simulink model "model"  (R2024a)
settings: Solver=FixedStepAuto  StartTime=0.0  StopTime=100  FixedStep=0.01  RelTol=1e-3
undefined symbols (not defined in the file or in its folder): e0_0, e1_0, e2_0, e3_0, q0, Thrust, vec
libraries: sharedtransform x21, sharedutil x4, aerolibsim3d x2, dspsigops x2, shared6dof x1, sim3dlib x1
(part 1 of 2)
settings Model: Creator=bemran  LastModifiedBy=bemran

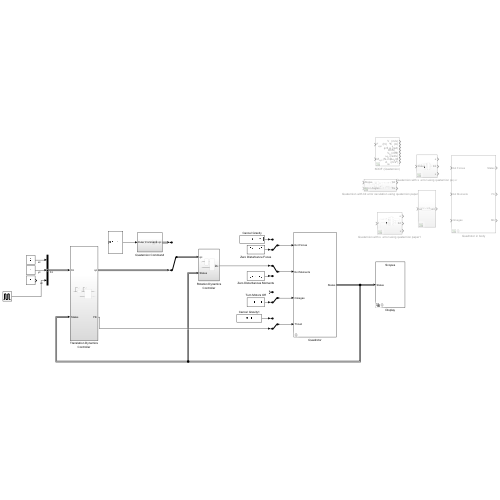
[thumbnail: Simulink's stored preview of the top-level diagram]
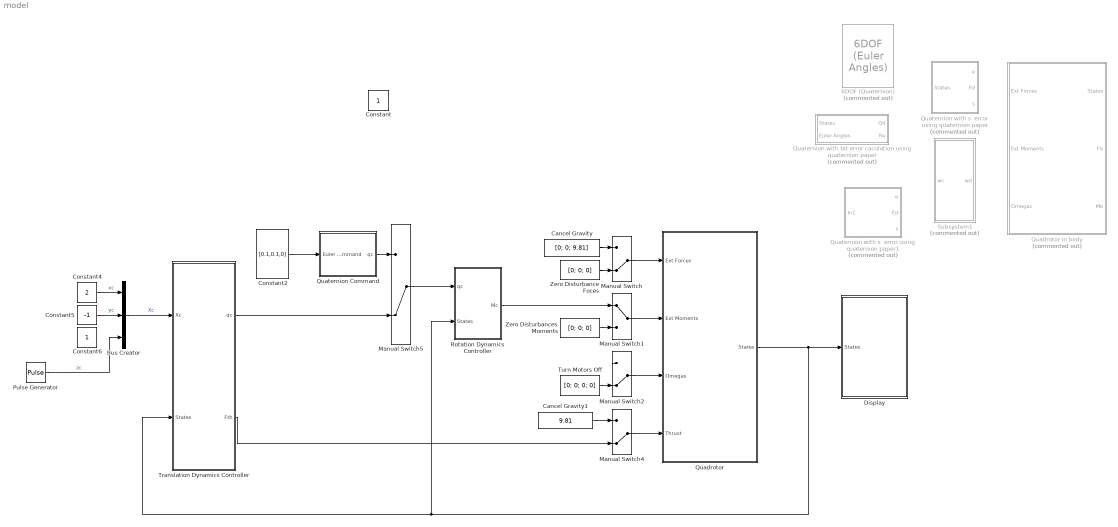
== system model ==
  6DOF (Quaternion) : shared6dof/6DOF (Euler Angles)  Commented=on  units=Metric (MKS)  mtype=Fixed  rep=Quaternion  xme_0=[0 0 0]  Vm_0=[0 0 0]  eul_0=[0 0 0]  pm_0=[0 0 0]  mass_0=1.0  mass_e=0.5  mass_f=2.0  inertia=eye(3)  inertia_e=eye(3)  inertia_f=2*eye(3)  k_quat=1.0  vre_flag=on  abi_flag=off  aMode=0  xme_statename=''  Vm_statename=''  eul_statename=''  quat_statename=''  pm_statename=''  mass_statename=''
      settings: LibrarySourceBlock=aerolib6dof2/6DOF (Quaternion)
  Bus Creator : BusCreator  Inputs=3
  Cancel Gravity : Constant  Value=[0; 0; 9.81]
  Cancel Gravity1 : Constant  Value=9.81
  Constant2 : Constant  Value=[0.1,0.1,0]
  Constant4 : Constant  Value=2
  Constant5 : Constant  Value=-1
  Constant6 : Constant
  Display : Subsystem  Variant=on  VariantControlMode=label  LabelModeActiveChoice=scopes  mask{VChoice=scopes}
      mask prompts: VChoice "Select method of display"
      mask init:
      | vssBlk = gcb;
      | choice = get_param(vssBlk,'VChoice');
      | if strcmp(choice,'animation')
      |     set_param(vssBlk, 'LabelModeActiveChoice', 'animation');
      | else
      |     set_param(vssBlk, 'LabelModeActiveChoice', 'scopes');
      | end
  Manual Switch{,2,4..5} (4 alike) : ManualSwitch  CurrentSetting=0
  Manual Switch1 : ManualSwitch
  Pulse Generator : DiscretePulseGenerator  PulseType=Time based  Amplitude=4  Period=20  PulseWidth=50
  Quadrotor : Subsystem  mask{VChoice=Thrust, mass=1, InertiaMatrix=eye(3)*0.1, thrust_coff=1, drag_coff=0.1, arm_length=0.3, VelocityBodyInitialValues=zeros(3,1), PositionReferenceInitialValues=zeros(3,1), OmegaInitialValues=zeros(3,1), EulerInitialValues=zeros(3,1)}
      mask prompts: VChoice "Select method of applying forces"; InertiaMatrix "Inertia Matrix"; thrust_coff "Thrust Coefficient"; drag_coff "Drag Coefficient"; arm_length "Arm Length"; VelocityBodyInitialValues "Velocity Body Initial Values"; PositionReferenceInitialValues "Position Reference Initial Values"; OmegaInitialValues "Omega Initial Values"; EulerInitialValues "Euler Initial Values"
      mask TypeOptions VChoice: Applied Forces in Body frame/VChoice
      mask TypeOptions mass: 6DOF NED Mixed/mass
      mask TypeOptions InertiaMatrix: 6DOF NED Mixed/InertiaMatrix
      mask TypeOptions thrust_coff: Mixer/thrust_coff
      mask TypeOptions drag_coff: Mixer/drag_coff
      mask TypeOptions arm_length: Mixer/arm_length
      mask TypeOptions VelocityBodyInitialValues: 6DOF NED Mixed/VelocityBodyInitialValues
      mask TypeOptions PositionReferenceInitialValues: 6DOF NED Mixed/PositionReferenceInitialValues
      mask TypeOptions OmegaInitialValues: 6DOF NED Mixed/OmegaInitialValues
      mask TypeOptions EulerInitialValues: 6DOF NED Mixed/EulerInitialValues
  Quadrotor in body : Subsystem  Commented=on  mask{VChoice=Thrust, mass=1, InertiaMatrix=eye(3)*0.1, thrust_coff=1, drag_coff=0.1, arm_length=0.3, VelocityBodyInitialValues=zeros(3,1), PositionReferenceInitialValues=zeros(3,1), OmegaInitialValues=zeros(3,1), EulerInitialValues=zeros(3,1)}
      mask prompts: VChoice "Select method of applying forces"; InertiaMatrix "Inertia Matrix"; thrust_coff "Thrust Coefficient"; drag_coff "Drag Coefficient"; arm_length "Arm Length"; VelocityBodyInitialValues "Velocity Body Initial Values"; PositionReferenceInitialValues "Position Reference Initial Values"; OmegaInitialValues "Omega Initial Values"; EulerInitialValues "Euler Initial Values"
      mask TypeOptions VChoice: Applied Forces in Body frame/VChoice
      mask TypeOptions mass: 6DOF NED Mixed/mass
      mask TypeOptions InertiaMatrix: 6DOF NED Mixed/InertiaMatrix
      mask TypeOptions thrust_coff: Mixer/thrust_coff
      mask TypeOptions drag_coff: Mixer/drag_coff
      mask TypeOptions arm_length: Mixer/arm_length
      mask TypeOptions VelocityBodyInitialValues: 6DOF NED Mixed/VelocityBodyInitialValues
      mask TypeOptions PositionReferenceInitialValues: 6DOF NED Mixed/PositionReferenceInitialValues
      mask TypeOptions OmegaInitialValues: 6DOF NED Mixed/OmegaInitialValues
      mask TypeOptions EulerInitialValues: 6DOF NED Mixed/EulerInitialValues
  Quaternion Command : Subsystem
  Quaternion with bit error caculation using quaternion paper : Subsystem  Commented=on
  Quaternion with s  error using quaternion paper : Subsystem  Commented=on
  Quaternion with s  error using quaternion paper1 : Subsystem  Commented=on
  Rotation Dynamics Controller : Subsystem
  Subsystem1 : Subsystem  Commented=on
  Translation Dynamics Controller : Subsystem
  Turn Motors Off : Constant  Value=[0; 0; 0; 0]
  Zero Disturbance Foces : Constant  Value=[0; 0; 0]
  Zero Disturbances Moments : Constant  Value=[0; 0; 0]
  Constant : Constant  IOType=siggen
  wires:
  Quadrotor/1(States) -> Translation Dynamics Controller/2(States), Rotation Dynamics Controller/2(States), Display/1(States)
  Zero Disturbance Foces/1 -> Manual Switch/2
  Manual Switch/1 -> Quadrotor/1(Ext Forces)
  Zero Disturbances Moments/1 -> Manual Switch1/2
  Manual Switch1/1 -> Quadrotor/2(Ext Moments)
  Manual Switch2/1 -> Quadrotor/3(Omegas)
  Turn Motors Off/1 -> Manual Switch2/2
  Constant4/1 -> Bus Creator/1  "xc"
  Pulse Generator/1 -> Bus Creator/3  "zc"
  Constant5/1 -> Bus Creator/2  "yc"
  Cancel Gravity/1 -> Manual Switch/1
  Manual Switch4/1 -> Quadrotor/4(Thrust)
  Cancel Gravity1/1 -> Manual Switch4/1
  Rotation Dynamics Controller/1(Mc) -> Manual Switch1/1
  Manual Switch5/1 -> Rotation Dynamics Controller/1(qc)
  Constant2/1 -> Quaternion Command/1(Euler Command)
  Quaternion Command/1(qc) -> Manual Switch5/1
  Bus Creator/1 -> Translation Dynamics Controller/1(Xc)  "Xc"
  Translation Dynamics Controller/1(qc) -> Manual Switch5/2
  Translation Dynamics Controller/2(Fth) -> Manual Switch4/2

== system model/Display ==
  States : Inport
  Animation : Subsystem  VariantControl=animation
  Scopes : Subsystem  VariantControl=scopes

== system model/Quadrotor ==
  Ext Forces : Inport
  Ext Moments : Inport  Port=2
  Omegas : Inport  Port=3
  Thrust : Inport  Port=4
  6DOF NED Mixed : Subsystem  mask{InertiaMatrix=InertiaMatrix, mass=mass, VelocityBodyInitialValues=VelocityBodyInitialValues, PositionReferenceInitialValues=PositionReferenceInitialValues, OmegaInitialValues=OmegaInitialValues, EulerInitialValues=EulerInitialValues}
      mask prompts: InertiaMatrix "Inertia Matrix"; VelocityBodyInitialValues "Velocity Body Initial Values"; PositionReferenceInitialValues "Position Reference Initial Values"; OmegaInitialValues "Omega Initial Values"; EulerInitialValues "Euler Initial Values"
      mask TypeOptions InertiaMatrix: Angular Velocity Dyanmics/InertiaMatrix
      mask TypeOptions mass: Translation Dynamics/mass
      mask TypeOptions VelocityBodyInitialValues: Translation Dynamics/VelocityBodyInitialValues
      mask TypeOptions PositionReferenceInitialValues: Translation Dynamics/PositionReferenceInitialValues
      mask TypeOptions OmegaInitialValues: Angular Velocity Dyanmics/OmegaInitialValues
      mask TypeOptions EulerInitialValues: Quaternion Dynamics/EulerInitialValues
      mask DialogControl Parameters Prompt: Parameters
      mask DialogControl Container6 Prompt: Initial Values
  Applied Forces in Body frame : Subsystem  Commented=on  Variant=on  VariantControlMode=label  LabelModeActiveChoice=Thrust  mask{VChoice=Thrust}
      mask prompts: VChoice "Select method of applying forces"
      mask Callback VChoice:
      | vssBlk = gcb;
      | choice = get_param(vssBlk,'VChoice');
      | if strcmp(choice,'Direct')
      |     set_param(vssBlk, 'LabelModeActiveChoice', 'Direct');
      | else
      |     set_param(vssBlk, 'LabelModeActiveChoice', 'Thrust');
      | end
  Bus Selector : BusSelector  OutputSignals=DCM_be
  Forces in Body frame : Subsystem  mask{mass=mass, Gravity=9.81}
  Forces in Body frame1 : Subsystem
  Mixer : Subsystem  mask{thrust_coff=thrust_coff, drag_coff=drag_coff, arm_length=arm_length}
      mask prompts: thrust_coff "Thrust Coefficient"; drag_coff "Drag Coefficient"; arm_length "Arm Length"
  States : Outport
  wires:
  6DOF NED Mixed/1(States) -> States/1, Bus Selector/1
  Forces in Body frame/1(Fe) -> [Fe], 6DOF NED Mixed/1(Fe)
  Bus Selector/1 -> Forces in Body frame/2(DCM_be)  "<DCM_be>"
  Omegas/1 -> Mixer/1(Omegas)
  Thrust/1 -> Forces in Body frame/3(Thrust)
  Mixer/2(Torques) -> Forces in Body frame1/2(Torque)
  Ext Moments/1 -> Forces in Body frame1/1(Ext Moments)
  Ext Forces/1 -> Forces in Body frame/1(Ext Forces)
  Forces in Body frame1/1(Mb) -> [Mb], 6DOF NED Mixed/2(Moments)

== system model/Quadrotor in body ==
  Ext Forces : Inport
  Ext Moments : Inport  Port=2
  Omegas : Inport  Port=3
  6DOF NED : Subsystem  mask{InertiaMatrix=InertiaMatrix, mass=mass, VelocityBodyInitialValues=VelocityBodyInitialValues, PositionReferenceInitialValues=PositionReferenceInitialValues, OmegaInitialValues=OmegaInitialValues, EulerInitialValues=EulerInitialValues}
      mask prompts: InertiaMatrix "Inertia Matrix"; VelocityBodyInitialValues "Velocity Body Initial Values"; PositionReferenceInitialValues "Position Reference Initial Values"; OmegaInitialValues "Omega Initial Values"; EulerInitialValues "Euler Initial Values"
      mask TypeOptions InertiaMatrix: Angular Velocity Dyanmics/InertiaMatrix
      mask TypeOptions mass: Translation Dynamics/mass
      mask TypeOptions VelocityBodyInitialValues: Translation Dynamics/VelocityBodyInitialValues
      mask TypeOptions PositionReferenceInitialValues: Translation Dynamics/PositionReferenceInitialValues
      mask TypeOptions OmegaInitialValues: Angular Velocity Dyanmics/OmegaInitialValues
      mask TypeOptions EulerInitialValues: Quaternion Dynamics/EulerInitialValues
      mask DialogControl Parameters Prompt: Parameters
      mask DialogControl Container6 Prompt: Initial Values
  Applied Forces in Body frame : Subsystem  Commented=on  Variant=on  VariantControlMode=label  LabelModeActiveChoice=Thrust  mask{VChoice=Thrust}
      mask prompts: VChoice "Select method of applying forces"
      mask Callback VChoice:
      | vssBlk = gcb;
      | choice = get_param(vssBlk,'VChoice');
      | if strcmp(choice,'Direct')
      |     set_param(vssBlk, 'LabelModeActiveChoice', 'Direct');
      | else
      |     set_param(vssBlk, 'LabelModeActiveChoice', 'Thrust');
      | end
  Bus Selector : BusSelector  OutputSignals=DCM_be
  Forces in Body frame : Subsystem  mask{mass=mass, Gain=9.81}
      mask prompts: Gain "Simulink:blkprm_prompts:GainGain"
      mask TypeOptions Gain:
      | Gravitational Force
      | in Body Frame/g/Gain
      mask DialogControl Gain Prompt: Gain:
  Forces in Body frame1 : Subsystem
  Mixer : Subsystem  mask{thrust_coff=thrust_coff, drag_coff=drag_coff, arm_length=arm_length}
      mask prompts: thrust_coff "Thrust Coefficient"; drag_coff "Drag Coefficient"; arm_length "Arm Length"
  States : Outport
  Fb : Outport  Port=2
  Mb : Outport  Port=3
  wires:
  Forces in Body frame1/1(Mb) -> 6DOF NED/2(Moments), Mb/1
  Ext Forces/1 -> Forces in Body frame/1(Ext Forces)
  Ext Moments/1 -> Forces in Body frame1/1(Ext Moments)
  Mixer/2(Torques) -> Forces in Body frame1/2(Torque)
  Mixer/1(Thrust) -> Forces in Body frame/3(Thrust)
  Omegas/1 -> Mixer/1(Omegas)
  Bus Selector/1 -> Forces in Body frame/2(DCM_be)  "<DCM_be>"
  Forces in Body frame/1(Fb) -> 6DOF NED/1(Fb), Fb/1
  6DOF NED/1(States) -> Bus Selector/1, States/1

== system model/Quaternion Command ==
  Euler Command : Inport
  Bus Creator1 : BusCreator  Inputs=q0,vec  OutDataTypeStr=Bus: QuaturnionBus
  Demux1 : Demux
  Mux1 : Mux  Inputs=3
  Rotation Angles to Quaternions : sharedtransform/Rotation Angles to Quaternions  rotationOrder=ZYX  aMode=aMode
  Selector : Selector  InputPortWidth=3  IndexOptions=Index vector (dialog)  Indices=[3 2 1]  OutputSizes=1
  qc : Outport  OutDataTypeStr=Bus: QuaturnionBus  PortDimensions=1
  wires:
  Selector/1 -> Rotation Angles to Quaternions/1
  Euler Command/1 -> Selector/1
  Demux1/3 -> Mux1/2
  Rotation Angles to Quaternions/1 -> Demux1/1
  Demux1/2 -> Mux1/1
  Demux1/4 -> Mux1/3
  Demux1/1 -> Bus Creator1/1  "q0"
  Mux1/1 -> Bus Creator1/2  "vec"
  Bus Creator1/1 -> qc/1  "q"

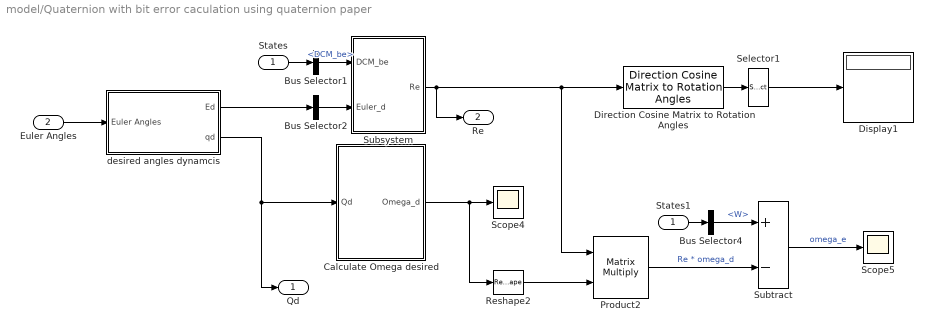
== system model/Quaternion with bit error caculation using quaternion paper ==
  States : Inport
  Euler Angles : Inport  Port=2
  Bus Selector1 : BusSelector  OutputSignals=DCM_be
  Bus Selector2 : BusSelector  OutputSignals=roll.rd,pitch.pd,yaw.yd  OutputAsBus=on
  Bus Selector4 : BusSelector  OutputSignals=W
  Calculate Omega desired : Subsystem
  Direction Cosine Matrix to Rotation Angles : sharedtransform/Direction Cosine Matrix to Rotation Angles  rotationOrder=ZYX  aMode=aMode  action=None  tolerance=eps(2)
      settings: LibrarySourceBlock=|
      | aerolibtransform2/Direction Cosine Matrix
      | to Rotation Angles
  Display1 : Display
  Product2 : Product  Multiplication=Matrix(*)
  Reshape2 : Reshape  OutputDimensionality=Column vector (2-D)
  Scope4 : Scope
  Scope5 : Scope
  Selector1 : Selector  InputPortWidth=3  IndexOptions=Index vector (dialog)  Indices=[3 2 1]  OutputSizes=1
  States1 : InportShadow
  Subsystem : Subsystem
  Subtract : Sum  Inputs=+-
  desired angles dynamcis : Subsystem
  Qd : Outport
  Re : Outport  Port=2
  wires:
  Subtract/1 -> Scope5/1  "omega_e"
  Direction Cosine Matrix to Rotation Angles/1 -> Selector1/1
  Bus Selector4/1 -> Subtract/1  "<W>"
  States/1 -> Bus Selector1/1
  Selector1/1 -> Display1/1
  Subsystem/1(Re) -> Product2/1, Direction Cosine Matrix to Rotation Angles/1, Re/1
  desired angles dynamcis/2(qd) -> Qd/1, Calculate Omega desired/1(Qd)
  desired angles dynamcis/1(Ed) -> Bus Selector2/1
  Product2/1 -> Subtract/2  "Re * omega_d"
  Bus Selector1/1 -> Subsystem/1(DCM_be)  "<DCM_be>"
  Reshape2/1 -> Product2/2
  Bus Selector2/1 -> Subsystem/2(Euler_d)
  Calculate Omega desired/1(Omega_d) -> Reshape2/1, Scope4/1
  Euler Angles/1 -> desired angles dynamcis/1(Euler Angles)
  States1/1 -> Bus Selector4/1

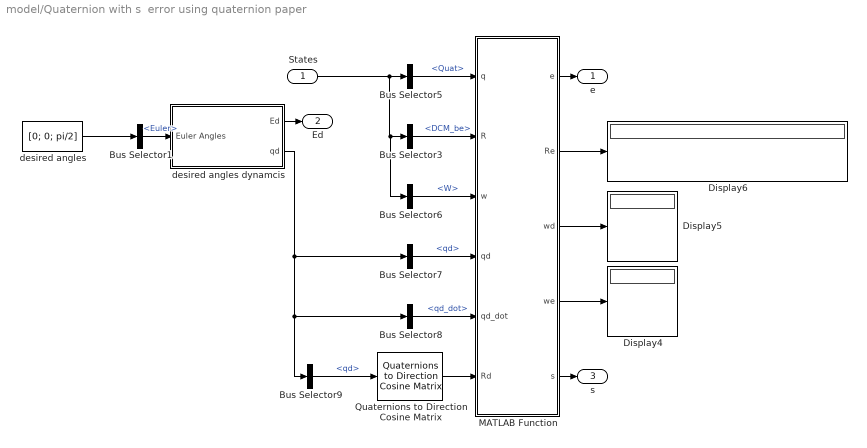
== system model/Quaternion with s  error using quaternion paper ==
  States : Inport
  Bus Selector1 : BusSelector  OutputSignals=Euler
  Bus Selector3 : BusSelector  OutputSignals=DCM_be
  Bus Selector5 : BusSelector  OutputSignals=Quat
  Bus Selector6 : BusSelector  OutputSignals=W
  Bus Selector7 : BusSelector  OutputSignals=qd
  Bus Selector8 : BusSelector  OutputSignals=qd_dot
  Bus Selector9 : BusSelector  OutputSignals=qd
  Display4 : Display
  Display5 : Display
  Display6 : Display
  MATLAB Function : MATLAB Function  TreatAsAtomicUnit=on
  Quaternions to Direction Cosine Matrix : sharedtransform/Quaternions to  Direction Cosine Matrix  aMode=aMode
      settings: LibrarySourceBlock=|
      | aerolibtransform2/Quaternions to
      | Direction Cosine Matrix
  desired angles : Constant  Value=[0; 0; pi/2]
  desired angles dynamcis : Subsystem
  e : Outport
  Ed : Outport  Port=2
  s : Outport  Port=3
  wires:
  Quaternions to Direction Cosine Matrix/1 -> MATLAB Function/6(Rd)
  MATLAB Function/2(Re) -> Display6/1
  MATLAB Function/4(we) -> Display4/1
  States/1 -> Bus Selector6/1, Bus Selector3/1, Bus Selector5/1
  desired angles/1 -> Bus Selector1/1
  desired angles dynamcis/2(qd) -> Bus Selector9/1, Bus Selector8/1, Bus Selector7/1
  Bus Selector1/1 -> desired angles dynamcis/1(Euler Angles)  "<Euler>"
  Bus Selector9/1 -> Quaternions to Direction Cosine Matrix/1  "<qd>"
  Bus Selector3/1 -> MATLAB Function/2(R)  "<DCM_be>"
  desired angles dynamcis/1(Ed) -> Ed/1
  Bus Selector7/1 -> MATLAB Function/4(qd)  "<qd>"
  Bus Selector6/1 -> MATLAB Function/3(w)  "<W>"
  Bus Selector8/1 -> MATLAB Function/5(qd_dot)  "<qd_dot>"
  Bus Selector5/1 -> MATLAB Function/1(q)  "<Quat>"
  MATLAB Function/3(wd) -> Display5/1
  MATLAB Function/5(s) -> s/1
  MATLAB Function/1(e) -> e/1

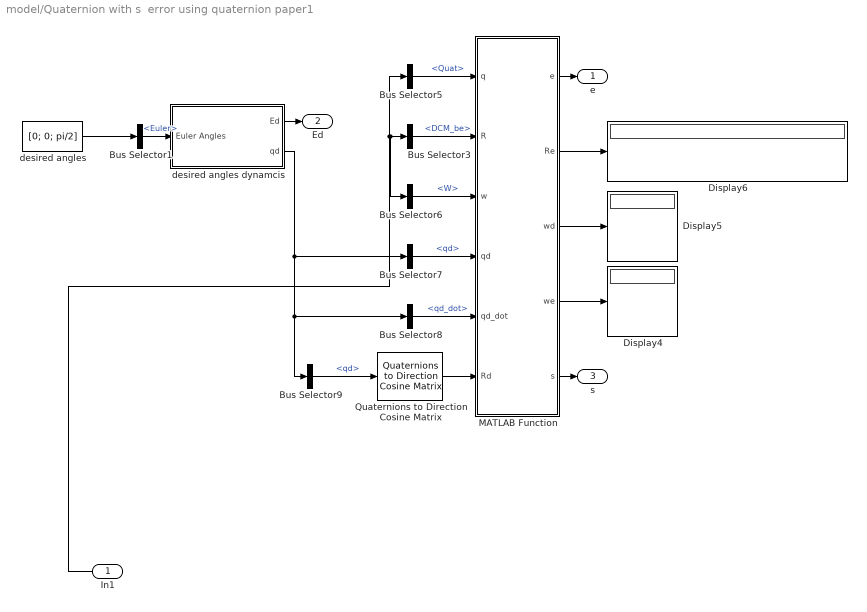
== system model/Quaternion with s  error using quaternion paper1 ==
  In1 : Inport
  Bus Selector1 : BusSelector  OutputSignals=Euler
  Bus Selector3 : BusSelector  OutputSignals=DCM_be
  Bus Selector5 : BusSelector  OutputSignals=Quat
  Bus Selector6 : BusSelector  OutputSignals=W
  Bus Selector7 : BusSelector  OutputSignals=qd
  Bus Selector8 : BusSelector  OutputSignals=qd_dot
  Bus Selector9 : BusSelector  OutputSignals=qd
  Display4 : Display
  Display5 : Display
  Display6 : Display
  MATLAB Function : MATLAB Function  TreatAsAtomicUnit=on
  Quaternions to Direction Cosine Matrix : sharedtransform/Quaternions to  Direction Cosine Matrix  aMode=aMode
      settings: LibrarySourceBlock=|
      | aerolibtransform2/Quaternions to
      | Direction Cosine Matrix
  desired angles : Constant  Value=[0; 0; pi/2]
  desired angles dynamcis : Subsystem
  e : Outport
  Ed : Outport  Port=2
  s : Outport  Port=3
  wires:
  Quaternions to Direction Cosine Matrix/1 -> MATLAB Function/6(Rd)
  MATLAB Function/2(Re) -> Display6/1
  MATLAB Function/4(we) -> Display4/1
  In1/1 -> Bus Selector5/1, Bus Selector6/1, Bus Selector3/1
  desired angles/1 -> Bus Selector1/1
  desired angles dynamcis/2(qd) -> Bus Selector9/1, Bus Selector8/1, Bus Selector7/1
  Bus Selector1/1 -> desired angles dynamcis/1(Euler Angles)  "<Euler>"
  Bus Selector9/1 -> Quaternions to Direction Cosine Matrix/1  "<qd>"
  Bus Selector3/1 -> MATLAB Function/2(R)  "<DCM_be>"
  desired angles dynamcis/1(Ed) -> Ed/1
  Bus Selector7/1 -> MATLAB Function/4(qd)  "<qd>"
  Bus Selector6/1 -> MATLAB Function/3(w)  "<W>"
  Bus Selector8/1 -> MATLAB Function/5(qd_dot)  "<qd_dot>"
  Bus Selector5/1 -> MATLAB Function/1(q)  "<Quat>"
  MATLAB Function/3(wd) -> Display5/1
  MATLAB Function/5(s) -> s/1
  MATLAB Function/1(e) -> e/1

== system model/Rotation Dynamics Controller ==
  qc : Inport  OutDataTypeStr=Bus: QuaturnionBus
  States : Inport  Port=2
  My paper controller : Subsystem
  Subsystem : Subsystem
  Mc : Outport
  wires:
  qc/1 -> Subsystem/1(qc)
  Subsystem/1(Rd) -> My paper controller/1(Rd)  "Rd"
  My paper controller/1(qw) -> Mc/1
  States/1 -> My paper controller/2(States)

== system model/Subsystem1 ==
  wc : Inport
  Add : Sum  Inputs=+-
  Bus Creator1 : BusCreator  Inputs=3
  Demux1 : Demux  Outputs=3
  Gain1 : Gain  Gain=1/10
  Integrator : Integrator  InitialCondition=[0,0,0]
  wd : Outport
  wires:
  Add/1 -> Gain1/1
  Bus Creator1/1 -> wd/1, Add/2  "wd"
  Integrator/1 -> Demux1/1
  Demux1/1 -> Bus Creator1/1  "pd"
  Demux1/3 -> Bus Creator1/3  "rd"
  Demux1/2 -> Bus Creator1/2  "qd"
  Gain1/1 -> Integrator/1
  wc/1 -> Add/1

== system model/Translation Dynamics Controller ==
  Xc : Inport
  States : Inport  Port=2
  My paper Translation Controller but for Quaternion : Subsystem
  desired position dynamcis : Subsystem
  qc : Outport  OutDataTypeStr=Bus: QuaturnionBus
  Fth : Outport  Port=2
  wires:
  desired position dynamcis/1(Xd) -> [Xd], My paper Translation Controller but for Quaternion/1(Xd)
  States/1 -> My paper Translation Controller but for Quaternion/2(States)
  My paper Translation Controller but for Quaternion/2(Fth) -> Fth/1
  Xc/1 -> [Xc], desired position dynamcis/1(Desired Position)
  My paper Translation Controller but for Quaternion/1(qc) -> qc/1

== system model/Display/Animation ==
  States : Inport
  Bus Selector : BusSelector  OutputSignals=Xe,Euler
  Simulation 3D Multirotor Pack : aerolibsim3d/Simulation 3D Multirotor Pack  Rotor1_T=off  Rotor1_R=off  Rotor2_T=off  Rotor2_R=off  Rotor3_T=off  Rotor3_R=off  Rotor4_T=off  Rotor4_R=off  Rotor5_T=off  Rotor5_R=off  Rotor6_T=off  Rotor6_R=off  Rotor7_T=off  Rotor7_R=off  Rotor8_T=off  Rotor8_R=off  Sensor1_T=off  Sensor1_R=off  Sensor2_T=off  Sensor2_R=off  GeoRadioButton=NED  AdjustForCesium=off  Heading0=90
  Simulation 3D Rotorcraft : aerolibsim3d/Simulation 3D Rotorcraft  Priority=-1  Mesh=Multirotor  MeshPath=/MathWorksAerospaceContent/Vehicles/Rotorcraft/Helicopter/Mesh/SK_Helicopter.SK_Helicopter  MeshPathLight=/MathWorksAerospaceContent/Vehicles/Rotorcraft/LightHelicopter/Mesh/SK_LightHelicopter.SK_LightHelicopter  MeshPathMulti=/MathWorksAerospaceContent/Vehicles/Rotorcraft/Multirotor/Mesh/SK_Quadcopter.SK_Quadcopter  AircraftColor=Red  ActorName=SimulinkVehicle3  Translation=zeros(11, 3)  Rotation=zeros(11, 3)  IsGHSensorEnabled=off  AreGHRaysVisible=on  IsOutputReshapeEnabled=off  GHRayLength=1524  GHBodyOffset=1.169  GHFrontTireRadius=0.196  GHLeftTireRadius=0.203  GHRightTireRadius=0.203  GHContactLocation1=[1.47 -1.04 1.169]  GHContactLocation2=[-1.24 -1.04 1.169]  GHContactLocation3=[-1.24 1.04 1.169]  GHContactLocation4=[1.47 1.04 1.169]  WoWSensorTolerance=0.05  LightsConfig=Automatic lights  LandingLightIntensity=300000  LandingLightConeAngle=15  LandingLightColor=[1 1 1]  HelicopterLeftLandingLightLocation=[0 0 0]  HelicopterLeftLandingLightOrientation=[0 0 0]  NoseLightIntensity=150000  NoseLightConeAngle=36  HelicopterNoseLightLocation=[0 0 0]  HelicopterNoseLightOrientation=[0 0 0]  NavLightIntensity=500  PositionLightIntensity=500  StrobeLightIntensity=5000  StrobeLightColor=[1 1 1]  StrobePeriod=1.5  StrobePulseWidth=6  BeaconLightIntensity=4000  BeaconLightColor=[1 0 0]  BeaconPeriod=1.5  BeaconPulseWidth=10  SampleTime=0.1  ActorType=SimulinkVehicle  ID=3  aMode=0  ActorTag=SimulinkVehicle3
  Simulation 3D Scene Configuration1 : sim3dlib/Simulation 3D Scene Configuration  Priority=0  ProjectFormat=Default Scenes  SceneDesc=Airport  ProjectName=C:\Program Files\MATLAB\R2024a\toolbox\shared\sim3d_projects\automotive_project_windows\UE\WindowsNoEditor\VehicleSimulation.exe  ScenePath=/Game/Maps/HwStrght  EnableOpenDRIVE=off  vehTagList={'Scene Origin';'SimulinkVehicle2';'SimulinkVehicle3'}  vehTag=SimulinkVehicle2  FreeCameraInitialTranslation=[-6, 0, 2]  FreeCameraDefaultInitialTranslation=[-6, 0, 2]  FreeCameraInitialRotation=[0, -15, 0]  FreeCameraDefaultInitialRotation=[0, -15, 0]  OpVisEn=off  Ts=.1  EnableWindow=on  EnableRemoteAccess=off  EnableWeather=off  SunAzimuth=90  SunAltitude=40.0  EnableGeospatialSun=off  Latitude=0  Longitude=0  Date=2023-01-01  Time=10:30:00  GeoTimeZone=-5.0  SunDaylightSaving=off  wind=1  clouds=10  EnableVolumetricClouds=off  CloudCoverage=0  CloudAltitude=6  fog=0  rain=0  RaindropsEffect=off  SnowDensity=0  EnableGeospatial=off  UseTrueOrigin=off  OriginHeight=200  OriginLatitude=40.744652  OriginLongitude=-73.988864  MapStyle=Aerial  AdditionalAssetIDs=[]  UseAdvancedSunSky=off  SolarTime=11  TimeZone=-5  Day=21  Month=9  Year=2022  UseDaylightSavingTime=on  DSTStartDay=10  DSTStartMonth=3  DSTEndDay=3  DSTEndMonth=11  DSTSwitchHour=2  sensorTag=MainCamera1  sensorId=1  sensorName=MainCamera1  mountLoc=Origin  offsetFlag=off  tmountOffset=[0, 0, 0]  rmountOffset=[0, 0, 0]  HorizontalResolution=1280  VerticalResolution=720  HorizontalFOV=60  mountPoint=[0 0 0]  mountOrientation=[0 0 0]  aMode=0  ID=1  GeoTrigger=Inactive
      settings: LibrarySourceBlock=aerolibsim3d/Simulation 3D Scene Configuration
  wires:
  Simulation 3D Multirotor Pack/1 -> Simulation 3D Rotorcraft/1
  Simulation 3D Multirotor Pack/2 -> Simulation 3D Rotorcraft/2
  Bus Selector/1 -> Simulation 3D Multirotor Pack/1  "<Xe>"
  Bus Selector/2 -> Simulation 3D Multirotor Pack/2  "<Euler>"
  States/1 -> Bus Selector/1

== system model/Display/Scopes ==
  States : Inport
  Bus Selector : BusSelector  OutputSignals=Xe,Euler
  Demux : Demux  Outputs=3
  Demux1 : Demux  Outputs=3
  Scope : Scope  NumInputPorts=3
  Scope1 : Scope  NumInputPorts=3
  wires:
  Demux/1 -> Scope/1
  Demux/2 -> Scope/2
  Demux/3 -> Scope/3
  Demux1/1 -> Scope1/1
  Demux1/2 -> Scope1/2
  Demux1/3 -> Scope1/3
  Bus Selector/2 -> Demux1/1  "<Euler>"
  Bus Selector/1 -> Demux/1  "<Xe>"
  States/1 -> Bus Selector/1

== system model/Quadrotor/6DOF NED Mixed ==
  Fe : Inport  OutDataTypeStr=double  Unit=N  PortDimensions=3
  Moments : Inport  Port=2  OutDataTypeStr=double
  Angular Velocity Dyanmics : Subsystem  mask{OmegaInitialValues=OmegaInitialValues, InertiaMatrix=InertiaMatrix}
      mask prompts: OmegaInitialValues "Omega Initial Values"; InertiaMatrix "Inertia Matrix"
  Quaternion Dynamics : Subsystem  mask{EulerInitialValues=EulerInitialValues}
      mask prompts: EulerInitialValues "Euler Initial Values"
  Translation Dynamics : Subsystem  mask{mass=mass, gravity=9.81, VelocityBodyInitialValues=VelocityBodyInitialValues, PositionReferenceInitialValues=PositionReferenceInitialValues}
      mask prompts: gravity "Gravity (m/s2)"; VelocityBodyInitialValues "Velocity Body Initial Values"; PositionReferenceInitialValues "Position Reference Initial Values"
  Bus Element Out : Outport  PortName=States  Element=Ae
  Bus Element Out1 : Outport  PortName=States  Element=Vb
  Bus Element Out2 : Outport  PortName=States  Element=Ve
  Bus Element Out3 : Outport  PortName=States  Element=Xe
  Bus Element Out4 : Outport  PortName=States  Element=DCM_be
  Bus Element Out5 : Outport  PortName=States  Element=Quat
  Bus Element Out6 : Outport  PortName=States  Element=Euler
  Bus Element Out7 : Outport  PortName=States  Element=W
  Bus Element Out8 : Outport  PortName=States  Element=Wdot
  wires:
  Quaternion Dynamics/1(DCM_be) -> Bus Element Out4/1, Translation Dynamics/2(DCM_be)
  Angular Velocity Dyanmics/2(Wdot) -> Bus Element Out8/1
  Quaternion Dynamics/2(Quat) -> Bus Element Out5/1
  Angular Velocity Dyanmics/1(W) -> Bus Element Out7/1, Quaternion Dynamics/1(w)
  Translation Dynamics/3(Ve) -> Bus Element Out2/1
  Moments/1 -> Angular Velocity Dyanmics/1(Moments)
  Quaternion Dynamics/3(Euler) -> Bus Element Out6/1
  Translation Dynamics/2(Vb) -> Bus Element Out1/1
  Translation Dynamics/4(Xe) -> Bus Element Out3/1
  Translation Dynamics/1(Ae) -> Bus Element Out/1
  Fe/1 -> Translation Dynamics/1(Fe)

== system model/Quadrotor/Applied Forces in Body frame ==
  Forces : Inport
  DCM_be : Inport  Port=2
  Apply Thrust and Gravitational Force : Subsystem  VariantControl=Thrust
  Direct Implementation to Body Forces : Subsystem  VariantControl=Direct
  Fb : Outport

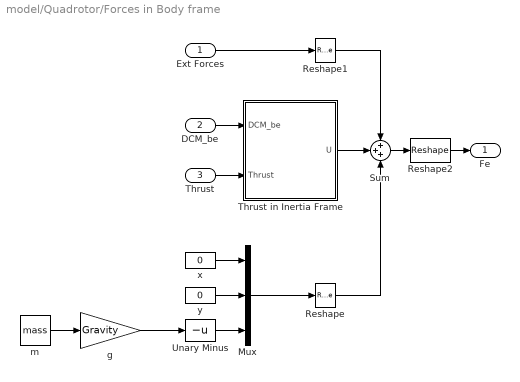
== system model/Quadrotor/Forces in Body frame ==
  Ext Forces : Inport
  DCM_be : Inport  Port=2
  Thrust : Inport  Port=3
  Mux : Mux  Inputs=3
  Reshape : Reshape  OutputDimensionality=Column vector (2-D)
  Reshape1 : Reshape  OutputDimensionality=Column vector (2-D)
  Reshape2 : Reshape
  Sum : Sum  Inputs=+++
  Thrust in Inertia Frame : Subsystem
  Unary Minus : UnaryMinus
  g : Gain  Gain=Gravity
  m : Constant  Value=mass
  x : Constant  Value=0
  y : Constant  Value=0
  Fe : Outport
  wires:
  Thrust in Inertia Frame/1(U) -> Sum/2
  Reshape1/1 -> Sum/1
  DCM_be/1 -> Thrust in Inertia Frame/1(DCM_be)
  Reshape/1 -> Sum/3
  Mux/1 -> Reshape/1
  Reshape2/1 -> Fe/1
  x/1 -> Mux/1
  y/1 -> Mux/2
  Ext Forces/1 -> Reshape1/1
  Sum/1 -> Reshape2/1
  m/1 -> g/1
  g/1 -> Unary Minus/1
  Thrust/1 -> Thrust in Inertia Frame/2(Thrust)
  Unary Minus/1 -> Mux/3

== system model/Quadrotor/Forces in Body frame1 ==
  Ext Moments : Inport
  Torque : Inport  Port=2
  Reshape2 : Reshape
  Sum : Sum  Inputs=+|+
  Mb : Outport
  wires:
  Ext Moments/1 -> Sum/1
  Reshape2/1 -> Mb/1
  Torque/1 -> Sum/2
  Sum/1 -> Reshape2/1

== system model/Quadrotor/Mixer ==
  Omegas : Inport
  Bus Creator : BusCreator  Inputs=3
  Fcn : Fcn  Expr=u(1) + u(2) + u(3) + u(4)
  Fcn1 : Fcn  Expr=-u(1) + u(3)
  Fcn2 : Fcn  Expr=-u(2) + u(4)
  Fcn3 : Fcn  Expr=u(1) - u(2) + u(3) - u(4)
  Square : Math  Operator=square
  b : Gain  Gain=thrust_coff
  c : Gain  Gain=drag_coff
  l : Gain  Gain=arm_length
  Thrust : Outport
  Torques : Outport  Port=2
  wires:
  b/1 -> Fcn/1, l/1
  l/1 -> Fcn2/1, Fcn1/1
  Omegas/1 -> Square/1
  c/1 -> Fcn3/1
  Fcn/1 -> Thrust/1
  Square/1 -> c/1, b/1
  Bus Creator/1 -> Torques/1
  Fcn1/1 -> Bus Creator/1  "Tx"
  Fcn2/1 -> Bus Creator/2  "Ty"
  Fcn3/1 -> Bus Creator/3  "Tz"

== system model/Quadrotor in body/6DOF NED ==
  Fb : Inport  OutDataTypeStr=double  Unit=N  PortDimensions=3
  Moments : Inport  Port=2  OutDataTypeStr=double
  Angular Velocity Dyanmics : Subsystem  mask{OmegaInitialValues=OmegaInitialValues, InertiaMatrix=InertiaMatrix}
      mask prompts: OmegaInitialValues "Omega Initial Values"; InertiaMatrix "Inertia Matrix"
  Quaternion Dynamics : Subsystem  mask{EulerInitialValues=EulerInitialValues}
      mask prompts: EulerInitialValues "Euler Initial Values"
  Translation Dynamics : Subsystem  mask{mass=mass, gravity=9.81, VelocityBodyInitialValues=VelocityBodyInitialValues, PositionReferenceInitialValues=PositionReferenceInitialValues}
      mask prompts: gravity "Gravity (m/s2)"; VelocityBodyInitialValues "Velocity Body Initial Values"; PositionReferenceInitialValues "Position Reference Initial Values"
  Bus Element Out : Outport  PortName=States  Element=Ab
  Bus Element Out1 : Outport  PortName=States  Element=Vb
  Bus Element Out2 : Outport  PortName=States  Element=Ve
  Bus Element Out3 : Outport  PortName=States  Element=Xe
  Bus Element Out4 : Outport  PortName=States  Element=DCM_be
  Bus Element Out5 : Outport  PortName=States  Element=Quat
  Bus Element Out6 : Outport  PortName=States  Element=Euler
  Bus Element Out7 : Outport  PortName=States  Element=W
  Bus Element Out8 : Outport  PortName=States  Element=Wdot
  wires:
  Fb/1 -> Translation Dynamics/1(Fb)
  Translation Dynamics/1(Ab) -> Bus Element Out/1
  Translation Dynamics/4(Xe) -> Bus Element Out3/1
  Translation Dynamics/2(Vb) -> Bus Element Out1/1
  Quaternion Dynamics/3(Euler) -> Bus Element Out6/1
  Moments/1 -> Angular Velocity Dyanmics/1(Moments)
  Translation Dynamics/3(Ve) -> Bus Element Out2/1
  Angular Velocity Dyanmics/1(W) -> Quaternion Dynamics/1(w), Bus Element Out7/1
  Quaternion Dynamics/2(Quat) -> Bus Element Out5/1
  Angular Velocity Dyanmics/2(Wdot) -> Bus Element Out8/1
  Quaternion Dynamics/1(DCM_be) -> Translation Dynamics/2(DCM_be), Bus Element Out4/1

== system model/Quadrotor in body/Applied Forces in Body frame ==
  Forces : Inport
  DCM_be : Inport  Port=2
  Apply Thrust and Gravitational Force : Subsystem  VariantControl=Thrust
  Direct Implementation to Body Forces : Subsystem  VariantControl=Direct
  Fb : Outport

== system model/Quadrotor in body/Forces in Body frame ==
  Ext Forces : Inport
  DCM_be : Inport  Port=2
  Thrust : Inport  Port=3
  Gravitational Force in Body Frame : Subsystem
  Mux : Mux  Inputs=3
  Reshape : Reshape  OutputDimensionality=Column vector (2-D)
  Reshape1 : Reshape  OutputDimensionality=Column vector (2-D)
  Reshape2 : Reshape
  Sum : Sum  Inputs=++-
  x : Constant  Value=0
  y : Constant  Value=0
  Fb : Outport
  wires:
  Reshape1/1 -> Sum/1
  Ext Forces/1 -> Reshape1/1
  y/1 -> Mux/2
  x/1 -> Mux/1
  Reshape2/1 -> Fb/1
  Mux/1 -> Reshape/1
  Reshape/1 -> Sum/3
  Thrust/1 -> Mux/3
  DCM_be/1 -> Gravitational Force in Body Frame/1(DCM_be)
  Sum/1 -> Reshape2/1
  Gravitational Force in Body Frame/1(FGb) -> Sum/2

== system model/Quadrotor in body/Forces in Body frame1 ==
  Ext Moments : Inport
  Torque : Inport  Port=2
  Reshape2 : Reshape
  Sum : Sum  Inputs=+|+
  Mb : Outport
  wires:
  Sum/1 -> Reshape2/1
  Torque/1 -> Sum/2
  Reshape2/1 -> Mb/1
  Ext Moments/1 -> Sum/1

== system model/Quadrotor in body/Mixer ==
  Omegas : Inport
  Bus Creator : BusCreator  Inputs=3
  Fcn : Fcn  Expr=u(1) + u(2) + u(3) + u(4)
  Fcn1 : Fcn  Expr=-u(1) + u(3)
  Fcn2 : Fcn  Expr=-u(2) + u(4)
  Fcn3 : Fcn  Expr=u(1) - u(2) + u(3) - u(4)
  Square : Math  Operator=square
  b : Gain  Gain=thrust_coff
  c : Gain  Gain=drag_coff
  l : Gain  Gain=arm_length
  Thrust : Outport
  Torques : Outport  Port=2
  wires:
  Fcn3/1 -> Bus Creator/3  "Tz"
  Fcn2/1 -> Bus Creator/2  "Ty"
  Fcn1/1 -> Bus Creator/1  "Tx"
  Bus Creator/1 -> Torques/1
  Square/1 -> b/1, c/1
  Fcn/1 -> Thrust/1
  c/1 -> Fcn3/1
  Omegas/1 -> Square/1
  l/1 -> Fcn1/1, Fcn2/1
  b/1 -> l/1, Fcn/1

== system model/Quaternion with bit error caculation using quaternion paper/Calculate Omega desired ==
  Qd : Inport
  Add : Sum
  Bus Selector : BusSelector  OutputSignals=qd.q0,qd.vec
  Bus Selector1 : BusSelector  OutputSignals=qd_dot.vec  OutputAsBus=on
  IdentityMatrix : IdentityMatrix  OutputDimensions=3
  Matrix Multiply : Product  Inputs=/*  Multiplication=Matrix(*)
  Product2 : Product
  Qd_dot : InportShadow
  Reshape1 : Reshape
  Reshape2 : Reshape  OutputDimensionality=Column vector (2-D)
  Skew Matrix : Subsystem
  Omega_d : Outport
  wires:
  Bus Selector1/1 -> Reshape2/1
  Skew Matrix/1(Out1) -> Add/2
  Add/1 -> Matrix Multiply/1
  Product2/1 -> Add/1
  Reshape2/1 -> Matrix Multiply/2
  IdentityMatrix/1 -> Product2/1
  Matrix Multiply/1 -> Reshape1/1
  Bus Selector/2 -> Skew Matrix/1(Inport)  "<vec>"
  Qd/1 -> Bus Selector/1
  Bus Selector/1 -> Product2/2  "<q0>"
  Qd_dot/1 -> Bus Selector1/1
  Reshape1/1 -> Omega_d/1

== system model/Quaternion with bit error caculation using quaternion paper/Subsystem ==
  DCM_be : Inport
  Euler_d : Inport  Port=2
  Matrix Multiply : Product  Multiplication=Matrix(*)
  Rotation Angles to Direction Cosine Matrix : sharedtransform/Rotation Angles to Direction Cosine Matrix  rotationOrder=ZYX  aMode=aMode
  Selector1 : Selector  InputPortWidth=3  IndexOptions=Index vector (dialog)  Indices=[3 2 1]  OutputSizes=1
  Transpose : Math  Operator=transpose
  Re : Outport
  wires:
  Selector1/1 -> Rotation Angles to Direction Cosine Matrix/1
  Rotation Angles to Direction Cosine Matrix/1 -> Transpose/1
  Euler_d/1 -> Selector1/1
  Matrix Multiply/1 -> Re/1
  DCM_be/1 -> Matrix Multiply/1
  Transpose/1 -> Matrix Multiply/2

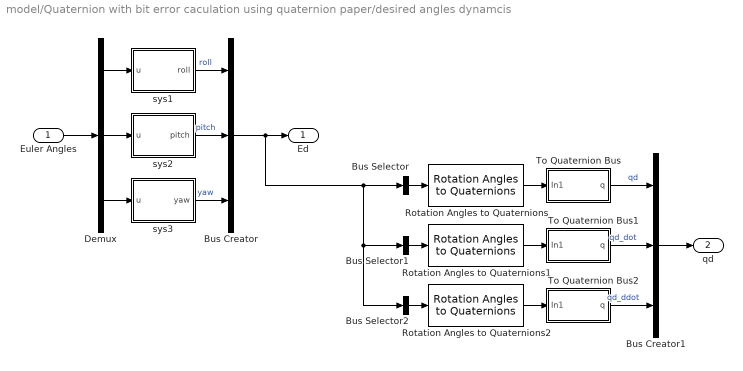
== system model/Quaternion with bit error caculation using quaternion paper/desired angles dynamcis ==
  Euler Angles : Inport
  Bus Creator : BusCreator  Inputs=3
  Bus Creator1 : BusCreator  Inputs=3
  Bus Selector : BusSelector  OutputSignals=yaw.yd,pitch.pd,roll.rd  OutputAsBus=on
  Bus Selector1 : BusSelector  OutputSignals=yaw.yd_dot,pitch.pd_dot,roll.rd_dot  OutputAsBus=on
  Bus Selector2 : BusSelector  OutputSignals=yaw.yd_ddot,pitch.pd_ddot,roll.rd_ddot  OutputAsBus=on
  Demux : Demux  Outputs=3
  Rotation Angles to Quaternions : sharedtransform/Rotation Angles to Quaternions  rotationOrder=ZYX  aMode=aMode
  Rotation Angles to Quaternions1 : sharedtransform/Rotation Angles to Quaternions  rotationOrder=ZYX  aMode=aMode
  Rotation Angles to Quaternions2 : sharedtransform/Rotation Angles to Quaternions  rotationOrder=ZYX  aMode=aMode
  To Quaternion Bus : Subsystem
  To Quaternion Bus1 : Subsystem
  To Quaternion Bus2 : Subsystem
  sys1 : Subsystem
  sys2 : Subsystem
  sys3 : Subsystem
  Ed : Outport
  qd : Outport  Port=2
  wires:
  sys2/1(pitch) -> Bus Creator/2  "pitch"
  Demux/3 -> sys3/1(u)
  Bus Creator/1 -> Bus Selector2/1, Bus Selector1/1, Bus Selector/1, Ed/1
  Demux/1 -> sys1/1(u)
  sys3/1(yaw) -> Bus Creator/3  "yaw"
  Euler Angles/1 -> Demux/1
  sys1/1(roll) -> Bus Creator/1  "roll"
  Demux/2 -> sys2/1(u)
  Bus Selector/1 -> Rotation Angles to Quaternions/1
  Bus Selector1/1 -> Rotation Angles to Quaternions1/1
  Bus Selector2/1 -> Rotation Angles to Quaternions2/1
  Rotation Angles to Quaternions/1 -> To Quaternion Bus/1(In1)
  Rotation Angles to Quaternions2/1 -> To Quaternion Bus2/1(In1)
  Rotation Angles to Quaternions1/1 -> To Quaternion Bus1/1(In1)
  To Quaternion Bus/1(q) -> Bus Creator1/1  "qd"
  To Quaternion Bus1/1(q) -> Bus Creator1/2  "qd_dot"
  To Quaternion Bus2/1(q) -> Bus Creator1/3  "qd_ddot"
  Bus Creator1/1 -> qd/1

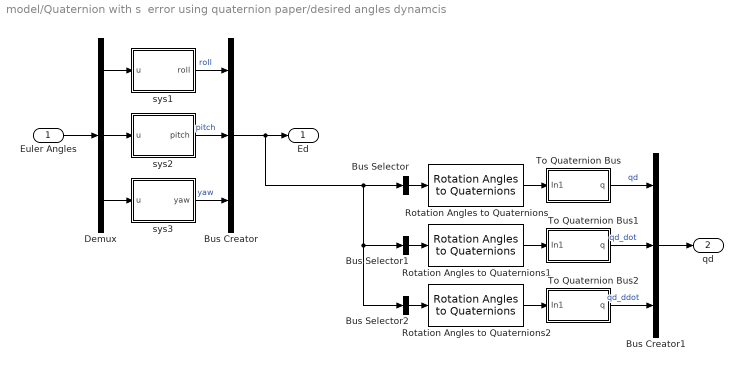
== system model/Quaternion with s  error using quaternion paper/desired angles dynamcis ==
  Euler Angles : Inport
  Bus Creator : BusCreator  Inputs=3
  Bus Creator1 : BusCreator  Inputs=3
  Bus Selector : BusSelector  OutputSignals=yaw.yd,pitch.pd,roll.rd  OutputAsBus=on
  Bus Selector1 : BusSelector  OutputSignals=yaw.yd_dot,pitch.pd_dot,roll.rd_dot  OutputAsBus=on
  Bus Selector2 : BusSelector  OutputSignals=yaw.yd_ddot,pitch.pd_ddot,roll.rd_ddot  OutputAsBus=on
  Demux : Demux  Outputs=3
  Rotation Angles to Quaternions : sharedtransform/Rotation Angles to Quaternions  rotationOrder=ZYX  aMode=aMode
  Rotation Angles to Quaternions1 : sharedtransform/Rotation Angles to Quaternions  rotationOrder=ZYX  aMode=aMode
  Rotation Angles to Quaternions2 : sharedtransform/Rotation Angles to Quaternions  rotationOrder=ZYX  aMode=aMode
  To Quaternion Bus : Subsystem
  To Quaternion Bus1 : Subsystem
  To Quaternion Bus2 : Subsystem
  sys1 : Subsystem
  sys2 : Subsystem
  sys3 : Subsystem
  Ed : Outport
  qd : Outport  Port=2
  wires:
  sys2/1(pitch) -> Bus Creator/2  "pitch"
  Demux/3 -> sys3/1(u)
  Bus Creator/1 -> Bus Selector2/1, Bus Selector1/1, Bus Selector/1, Ed/1
  Demux/1 -> sys1/1(u)
  sys3/1(yaw) -> Bus Creator/3  "yaw"
  Euler Angles/1 -> Demux/1
  sys1/1(roll) -> Bus Creator/1  "roll"
  Demux/2 -> sys2/1(u)
  Bus Selector/1 -> Rotation Angles to Quaternions/1
  Bus Selector1/1 -> Rotation Angles to Quaternions1/1
  Bus Selector2/1 -> Rotation Angles to Quaternions2/1
  Rotation Angles to Quaternions/1 -> To Quaternion Bus/1(In1)
  Rotation Angles to Quaternions2/1 -> To Quaternion Bus2/1(In1)
  Rotation Angles to Quaternions1/1 -> To Quaternion Bus1/1(In1)
  To Quaternion Bus/1(q) -> Bus Creator1/1  "qd"
  To Quaternion Bus1/1(q) -> Bus Creator1/2  "qd_dot"
  To Quaternion Bus2/1(q) -> Bus Creator1/3  "qd_ddot"
  Bus Creator1/1 -> qd/1

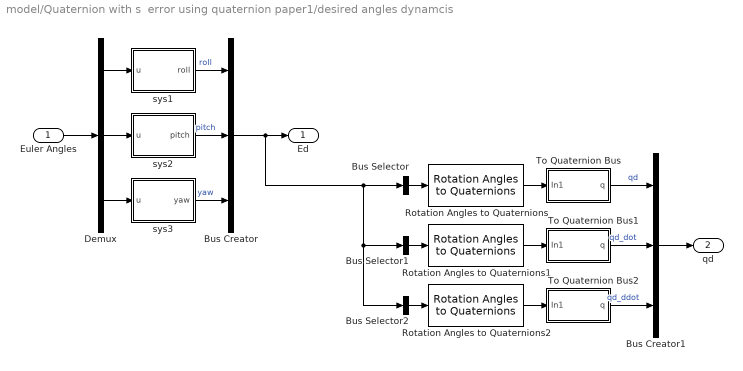
== system model/Quaternion with s  error using quaternion paper1/desired angles dynamcis ==
  Euler Angles : Inport
  Bus Creator : BusCreator  Inputs=3
  Bus Creator1 : BusCreator  Inputs=3
  Bus Selector : BusSelector  OutputSignals=yaw.yd,pitch.pd,roll.rd  OutputAsBus=on
  Bus Selector1 : BusSelector  OutputSignals=yaw.yd_dot,pitch.pd_dot,roll.rd_dot  OutputAsBus=on
  Bus Selector2 : BusSelector  OutputSignals=yaw.yd_ddot,pitch.pd_ddot,roll.rd_ddot  OutputAsBus=on
  Demux : Demux  Outputs=3
  Rotation Angles to Quaternions : sharedtransform/Rotation Angles to Quaternions  rotationOrder=ZYX  aMode=aMode
  Rotation Angles to Quaternions1 : sharedtransform/Rotation Angles to Quaternions  rotationOrder=ZYX  aMode=aMode
  Rotation Angles to Quaternions2 : sharedtransform/Rotation Angles to Quaternions  rotationOrder=ZYX  aMode=aMode
  To Quaternion Bus : Subsystem
  To Quaternion Bus1 : Subsystem
  To Quaternion Bus2 : Subsystem
  sys1 : Subsystem
  sys2 : Subsystem
  sys3 : Subsystem
  Ed : Outport
  qd : Outport  Port=2
  wires:
  sys2/1(pitch) -> Bus Creator/2  "pitch"
  Demux/3 -> sys3/1(u)
  Bus Creator/1 -> Bus Selector2/1, Bus Selector1/1, Bus Selector/1, Ed/1
  Demux/1 -> sys1/1(u)
  sys3/1(yaw) -> Bus Creator/3  "yaw"
  Euler Angles/1 -> Demux/1
  sys1/1(roll) -> Bus Creator/1  "roll"
  Demux/2 -> sys2/1(u)
  Bus Selector/1 -> Rotation Angles to Quaternions/1
  Bus Selector1/1 -> Rotation Angles to Quaternions1/1
  Bus Selector2/1 -> Rotation Angles to Quaternions2/1
  Rotation Angles to Quaternions/1 -> To Quaternion Bus/1(In1)
  Rotation Angles to Quaternions2/1 -> To Quaternion Bus2/1(In1)
  Rotation Angles to Quaternions1/1 -> To Quaternion Bus1/1(In1)
  To Quaternion Bus/1(q) -> Bus Creator1/1  "qd"
  To Quaternion Bus1/1(q) -> Bus Creator1/2  "qd_dot"
  To Quaternion Bus2/1(q) -> Bus Creator1/3  "qd_ddot"
  Bus Creator1/1 -> qd/1

== system model/Rotation Dynamics Controller/My paper controller ==
  Rd : Inport
  States : Inport  Port=2
  Bus Selector1 : BusSelector  OutputSignals=DCM_be,W
  Constant1 : Constant  Value=eye(3) * 14
  Constant2 : Constant  Value=eye(3) * 15
  Inertia Matrix : Constant  Value=eye(3)*0.1
  Integrator : Integrator  InitialCondition=[0;0;0]
  MATLAB Function : MATLAB Function  TreatAsAtomicUnit=on
  Product2 : Product  Inputs=**  Multiplication=Matrix(*)  SaturateOnIntegerOverflow=on  OutDataTypeStr=Inherit: Same as first input
  qw : Outport
  wires:
  Bus Selector1/1 -> MATLAB Function/3(R)  "<DCM_be>"
  Constant2/1 -> MATLAB Function/2(Kw)
  Bus Selector1/2 -> MATLAB Function/4(w)  "<W>"
  MATLAB Function/2(sw) -> [sw]
  Rd/1 -> MATLAB Function/5(Rd)
  MATLAB Function/1(sr) -> [sr]
  Constant1/1 -> MATLAB Function/1(Kr)
  MATLAB Function/5(wd_dot) -> Integrator/1
  MATLAB Function/3(wc) -> [wc]
  States/1 -> Bus Selector1/1
  Integrator/1 -> MATLAB Function/6(wd)
  MATLAB Function/4(qw) -> Product2/2
  Inertia Matrix/1 -> Product2/1
  Product2/1 -> qw/1  "Mc"

== system model/Rotation Dynamics Controller/Subsystem ==
  qc : Inport  OutDataTypeStr=Bus: QuaturnionBus
  Add1 : Sum  Inputs=+-
  Bus Creator2 : BusCreator  Inputs=q0,vec  OutDataTypeStr=Bus: QuaturnionBus
  Bus Selector : BusSelector  OutputSignals=q0,vec  OutputAsBus=on
  Demux2 : Demux
  Gain2 : Gain  Gain=50
  Integrator1 : Integrator  InitialCondition=[1;0;0;0]
  Mux : Mux  Inputs=3
  Quaternions to Direction Cosine Matrix : sharedtransform/Quaternions to  Direction Cosine Matrix  aMode=aMode
      settings: LibrarySourceBlock=|
      | aerolibtransform2/Quaternions to
      | Direction Cosine Matrix
  Reshape : Reshape  OutputDimensionality=Column vector (2-D)
  Rd : Outport
  wires:
  Demux2/3 -> Mux/2
  Demux2/2 -> Mux/1
  Gain2/1 -> Integrator1/1
  Demux2/4 -> Mux/3
  Demux2/1 -> Bus Creator2/1  "q0"
  Mux/1 -> Bus Creator2/2  "vec"
  Quaternions to Direction Cosine Matrix/1 -> Rd/1
  Bus Creator2/1 -> [qd]  "q"
  Integrator1/1 -> Demux2/1, Quaternions to Direction Cosine Matrix/1, Add1/2
  Add1/1 -> Gain2/1
  qc/1 -> [qc], Bus Selector/1
  Reshape/1 -> Add1/1
  Bus Selector/1 -> Reshape/1

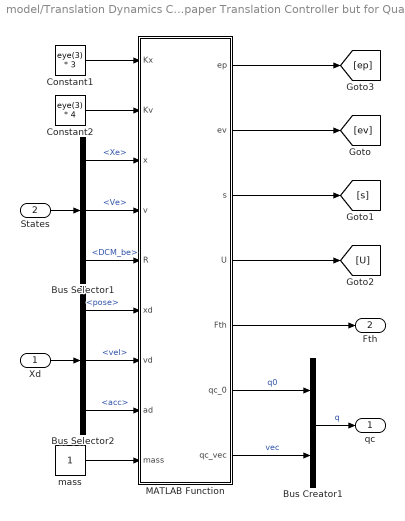
== system model/Translation Dynamics Controller/My paper Translation Controller but for Quaternion ==
  Xd : Inport
  States : Inport  Port=2
  Bus Creator1 : BusCreator  Inputs=q0,vec  OutDataTypeStr=Bus: QuaturnionBus
  Bus Selector1 : BusSelector  OutputSignals=Xe,Ve,DCM_be
  Bus Selector2 : BusSelector  OutputSignals=pose,vel,acc
  Constant1 : Constant  Value=eye(3) * 3
  Constant2 : Constant  Value=eye(3) * 4
  MATLAB Function : MATLAB Function  TreatAsAtomicUnit=on
  mass : Constant
  qc : Outport  OutDataTypeStr=Bus: QuaturnionBus  PortDimensions=1
  Fth : Outport  Port=2
  wires:
  States/1 -> Bus Selector1/1
  Constant1/1 -> MATLAB Function/1(Kx)
  Bus Selector1/2 -> MATLAB Function/4(v)  "<Ve>"
  Constant2/1 -> MATLAB Function/2(Kv)
  Bus Selector1/1 -> MATLAB Function/3(x)  "<Xe>"
  mass/1 -> MATLAB Function/9(mass)
  Xd/1 -> Bus Selector2/1
  Bus Selector2/2 -> MATLAB Function/7(vd)  "<vel>"
  Bus Selector2/1 -> MATLAB Function/6(xd)  "<pose>"
  Bus Selector2/3 -> MATLAB Function/8(ad)  "<acc>"
  MATLAB Function/5(Fth) -> Fth/1
  Bus Selector1/3 -> MATLAB Function/5(R)  "<DCM_be>"
  MATLAB Function/1(ep) -> [ep]
  MATLAB Function/2(ev) -> [ev]
  MATLAB Function/3(s) -> [s]
  MATLAB Function/4(U) -> [U]
  Bus Creator1/1 -> qc/1  "q"
  MATLAB Function/7(qc_vec) -> Bus Creator1/2  "vec"
  MATLAB Function/6(qc_0) -> Bus Creator1/1  "q0"

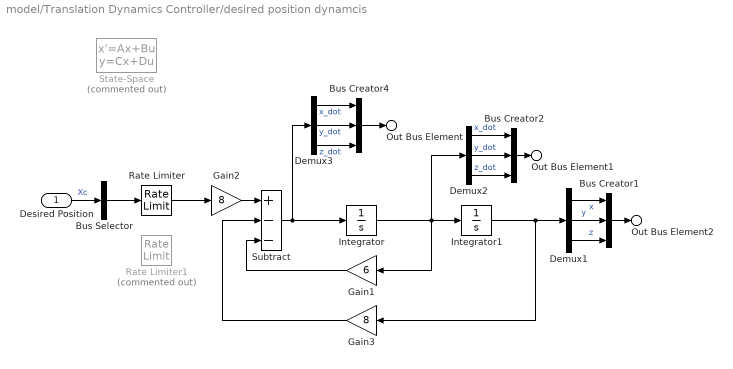
== system model/Translation Dynamics Controller/desired position dynamcis ==
  Desired Position : Inport
  Bus Creator1 : BusCreator  Inputs=3
  Bus Creator2 : BusCreator  Inputs=3
  Bus Creator4 : BusCreator  Inputs=3
  Bus Selector : BusSelector  OutputSignals=xc,yc,zc  OutputAsBus=on
  Demux1 : Demux  Outputs=3
  Demux2 : Demux  Outputs=3
  Demux3 : Demux  Outputs=3
  Gain1 : Gain  Gain=6
  Gain2 : Gain  Gain=8
  Gain3 : Gain  Gain=8
  Integrator : Integrator  InitialCondition=[0;0;0]
  Integrator1 : Integrator  InitialCondition=[0;0;0]
  Rate Limiter : RateLimiter  RisingSlewLimit=[1;1;1]*3  FallingSlewLimit=[-1;-1;-1]*3  SampleTimeMode=inherited
  Rate Limiter1 : RateLimiter  Commented=on  RisingSlewLimit=[1;1;10]  FallingSlewLimit=[-1;-1;-10]  SampleTimeMode=inherited
  State-Space : StateSpace  Commented=on  A="[0 0 0 1 0 0 ; 0 0 0 0 1 0; 0 0 0 0 0 1; -8  0 0 -6 0 0; 0 -8 0 0 -6 0; 0 0 -8 0 0 -6]"  B=[zeros(3,3); eye(3) * 8]  C=eye(6)  D=zeros(6,3)  InitialCondition=0
  Subtract : Sum  Inputs=+--
  Out Bus Element2 : Outport  PortName=Xd  Element=pose
  Out Bus Element1 : Outport  PortName=Xd  Element=vel
  Out Bus Element : Outport  PortName=Xd  Element=acc
  wires:
  Bus Creator1/1 -> Out Bus Element2/1
  Bus Selector/1 -> Rate Limiter/1
  Bus Creator2/1 -> Out Bus Element1/1
  Demux1/3 -> Bus Creator1/3  "z"
  Demux2/2 -> Bus Creator2/2  "y_dot"
  Demux2/3 -> Bus Creator2/3  "z_dot"
  Demux2/1 -> Bus Creator2/1  "x_dot"
  Demux1/1 -> Bus Creator1/1  "x"
  Demux1/2 -> Bus Creator1/2  "y"
  Desired Position/1 -> Bus Selector/1  "Xc"
  Subtract/1 -> Demux3/1, Integrator/1
  Integrator/1 -> Demux2/1, Integrator1/1, Gain1/1
  Integrator1/1 -> Gain3/1, Demux1/1
  Gain1/1 -> Subtract/3
  Gain2/1 -> Subtract/1
  Demux3/1 -> Bus Creator4/1  "x_dot"
  Demux3/2 -> Bus Creator4/2  "y_dot"
  Demux3/3 -> Bus Creator4/3  "z_dot"
  Bus Creator4/1 -> Out Bus Element/1
  Gain3/1 -> Subtract/2
  Rate Limiter/1 -> Gain2/1

== system model/Quadrotor/6DOF NED Mixed/Angular Velocity Dyanmics ==
  Moments : Inport  OutDataTypeStr=double
  Bus Creator1 : BusCreator  Inputs=3
  Bus Creator2 : BusCreator  Inputs=3
  Centrifugal Moments : Subsystem
  Demux1 : Demux  Outputs=3
  Demux2 : Demux  Outputs=3
  Inertia Matrix : Constant  Value=InertiaMatrix
  Product2 : Product  Inputs=*/  Multiplication=Matrix(*)  SaturateOnIntegerOverflow=on  OutDataTypeStr=Inherit: Same as first input
  Reshape : Reshape
  Reshape1 : Reshape  OutputDimensionality=Row vector (2-D)
  Sum2 : Sum  Inputs=++|  SaturateOnIntegerOverflow=on
  Wdot Integ : Integrator  InitialCondition=OmegaInitialValues  ContinuousStateAttributes={'p', 'q', 'r'}
  W : Outport
  Wdot : Outport  Port=2  OutDataTypeStr=double  Unit=rad/s^2  VectorParamsAs1DForOutWhenUnconnected=off
  wires:
  Product2/1 -> Reshape/1
  Centrifugal Moments/1((I * w) x w) -> Sum2/2
  Inertia Matrix/1 -> Product2/2
  Moments/1 -> Sum2/1
  Reshape1/1 -> Product2/1
  Demux1/1 -> Bus Creator1/1  "p"
  Wdot Integ/1 -> Demux1/1
  Demux1/3 -> Bus Creator1/3  "r"
  Demux1/2 -> Bus Creator1/2  "q"
  Bus Creator1/1 -> W/1, Centrifugal Moments/1(w)  "W"
  Sum2/1 -> Reshape1/1
  Reshape/1 -> Demux2/1, Wdot Integ/1
  Demux2/2 -> Bus Creator2/2  "qdot"
  Demux2/3 -> Bus Creator2/3  "rdot"
  Demux2/1 -> Bus Creator2/1  "pdot"
  Bus Creator2/1 -> Wdot/1  "Wdot"

== system model/Quadrotor/6DOF NED Mixed/Quaternion Dynamics ==
  w : Inport
  Integrating : Subsystem
  Mux : Mux  Inputs=2
  Quat to Euler : Subsystem
  Quaternions to Direction Cosine Matrix : sharedtransform/Quaternions to  Direction Cosine Matrix  aMode=aMode
  q0_dot : Subsystem
  qvec_dot : Subsystem
  DCM_be : Outport  OutDataTypeStr=double  VectorParamsAs1DForOutWhenUnconnected=off
  Quat : Outport  Port=2  OutDataTypeStr=double  VectorParamsAs1DForOutWhenUnconnected=off
  Euler : Outport  Port=3  OutDataTypeStr=double  VectorParamsAs1DForOutWhenUnconnected=off
  wires:
  Integrating/1(Quat) -> Quat/1, Quaternions to Direction Cosine Matrix/1, Quat to Euler/1(q), q0_dot/2(q), qvec_dot/2(q)
  qvec_dot/1(qvec_dot) -> Mux/2
  q0_dot/1(q0_dot) -> Mux/1
  Quaternions to Direction Cosine Matrix/1 -> DCM_be/1
  w/1 -> qvec_dot/1(w), q0_dot/1(w)
  Mux/1 -> Integrating/1(qdot)
  Quat to Euler/1(euler) -> Euler/1

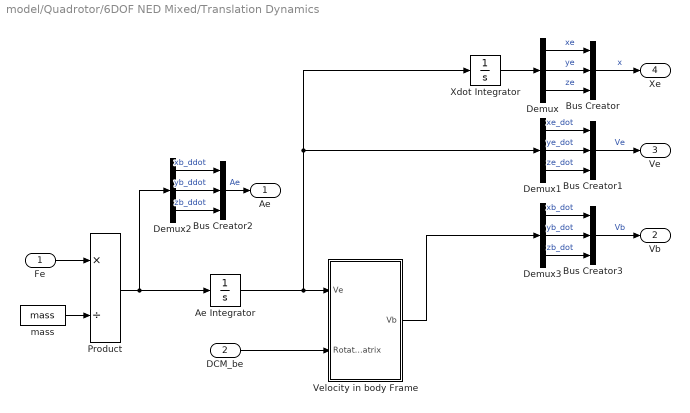
== system model/Quadrotor/6DOF NED Mixed/Translation Dynamics ==
  Fe : Inport
  DCM_be : Inport  Port=2
  Ae Integrator : Integrator  InitialCondition=VelocityBodyInitialValues  ContinuousStateAttributes={'u', 'v', 'w'}
  Bus Creator{,1..3} (4 alike) : BusCreator  Inputs=3
  Demux{,1..3} (4 alike) : Demux  Outputs=3
  Product : Product  Inputs=*/
  Velocity in body Frame : Subsystem
  Xdot Integrator : Integrator  InitialCondition=PositionReferenceInitialValues  ContinuousStateAttributes={'xr', 'ye', 'ze'}
  mass : Constant  Value=mass
  Ae : Outport  OutDataTypeStr=double  Unit=m/s^2  VectorParamsAs1DForOutWhenUnconnected=off
  Vb : Outport  Port=2  OutDataTypeStr=double  Unit=m/s  VectorParamsAs1DForOutWhenUnconnected=off
  Ve : Outport  Port=3  OutDataTypeStr=double  Unit=m/s  VectorParamsAs1DForOutWhenUnconnected=off
  Xe : Outport  Port=4
  wires:
  mass/1 -> Product/2
  Demux/2 -> Bus Creator/2  "ye"
  Demux1/2 -> Bus Creator1/2  "ye_dot"
  Bus Creator/1 -> Xe/1  "x"
  Demux/1 -> Bus Creator/1  "xe"
  Xdot Integrator/1 -> Demux/1
  Demux/3 -> Bus Creator/3  "ze"
  Demux1/3 -> Bus Creator1/3  "ze_dot"
  Demux1/1 -> Bus Creator1/1  "xe_dot"
  DCM_be/1 -> Velocity in body Frame/2(Rotation Matrix)
  Ae Integrator/1 -> Demux1/1, Xdot Integrator/1, Velocity in body Frame/1(Ve)
  Velocity in body Frame/1(Vb) -> Demux3/1
  Demux2/3 -> Bus Creator2/3  "zb_ddot"
  Bus Creator2/1 -> Ae/1  "Ae"
  Demux2/2 -> Bus Creator2/2  "yb_ddot"
  Demux2/1 -> Bus Creator2/1  "xb_ddot"
  Bus Creator1/1 -> Ve/1  "Ve"
  Demux3/1 -> Bus Creator3/1  "xb_dot"
  Demux3/3 -> Bus Creator3/3  "zb_dot"
  Demux3/2 -> Bus Creator3/2  "yb_dot"
  Bus Creator3/1 -> Vb/1  "Vb"
  Product/1 -> Ae Integrator/1, Demux2/1
  Fe/1 -> Product/1

== system model/Quadrotor/Applied Forces in Body frame/Apply Thrust and Gravitational Force ==
  Forces : Inport
  DCM_be : Inport  Port=2
  Forces in Body frame : Subsystem  mask{mass=mass, Gain=9.81}
      mask prompts: Gain "Simulink:blkprm_prompts:GainGain"
      mask TypeOptions Gain:
      | Gravitational Force
      | in Body Frame/g/Gain
      mask DialogControl Gain Prompt: Gain:
  Fb : Outport
  wires:
  Forces in Body frame/1(Fb) -> Fb/1
  DCM_be/1 -> Forces in Body frame/2(DCM_be)
  Forces/1 -> Forces in Body frame/1(Thrust)

== system model/Quadrotor/Applied Forces in Body frame/Direct Implementation to Body Forces ==
  Forces : Inport
  DCM_be : Inport  Port=2
  Terminator3 : Terminator
  Fb : Outport
  wires:
  Forces/1 -> Fb/1
  DCM_be/1 -> Terminator3/1
